simulink library "AeroLib"  (Simulink 6.0)
settings: Solver=ode45  SolverMode=SingleTasking  StartTime=0.0  StopTime=10.0  RelTol=1e-3
undefined symbols (not defined in the file): Aero, Ap, Atm, Control, Controls, Eng, Flight_cg, Flight_DamperON, Flight_delta_isa, Flight_DeltaSpiral, Flight_InertiaSelect, Flight_ixx, Flight_ixz, Flight_iyy, Flight_izz, Flight_latitude, Flight_LoiterLenght, Flight_LoiterMode, Flight_LoiterRadius, Flight_longitude, Flight_MaxTargetPoints, Flight_SensorsON, Flight_TimeStep, Flight_TowerWind_X, Flight_TowerWind_Y, Flight_TowerWind_Z, Flight_TowerWindON, Flight_Trimming, Flight_TurbON, Flight_weight, Flight_WindGustON, Flight_WindShearON, Flight_ycg, Flight_zcg, Geom, Lgear, Mass, PEG_CDwbnp, PEG_CLht, PEG_CLht_elev, PEG_CLwbnp, PEG_CMht, PEG_CMwbnp, PEG_CNbeta, PEG_CNr, PEG_CNrud, PEG_CRail, PEG_CRbeta, PEG_CRp, PEG_CRrud, PEG_CYbeta, PEG_CYrud, pow, Sensors
libraries: AeroLib x133, simulink3 x49, simulink x37, aerospace x11
(part 2 of 7)

== system AeroLib/AtmosphericData/Simple_Wind_Gust ==
  note: Horizontal wind direction 0 deg ==> North
      | Horizontal wind direction 90 deg ==> East
      | Horizontal wind direction 180 deg ==> South
      | Horizontal wind direction 270 deg ==> West
      |
      |
      |
      |
      |
      |
      |
      |
      |
      |
      |
      |
      |
      |
      |
      | Vertical wind speed negative ==> Up (ft/s)
      | Vertical wind speed positive ==> Down (ft/s)
  From_Reset : Inport  Port=1  LatchInput=off
  From_Inputs : Inport  Port=2  LatchInput=off
  Band-Limited White Noise : simulink3/Sources/Band-Limited White Noise  Cov=[0.1]  Ts=Flight_TimeStep  seed=[23341]
  Bus Selector : BusSelector  DialogController=Simulink.DDGSource_Bus  OutputSignals=Horiz_Wind_Speed,Horiz_Wind_Dir,Vert_Wind_Speed
  Constant2 : Constant  Value=Flight_WindGustON
  Deg-->Rad : Gain  Gain=pi/180  SaturateOnIntegerOverflow=on
  Demux : Demux  Outputs=2
  Gain : Gain  Gain=Wgain  SaturateOnIntegerOverflow=on
  Mux : Mux  Inputs=2
  Mux1 : Mux  Inputs=3
  Product : Product  SaturateOnIntegerOverflow=on  InputSameDT=on
  Product1 : Product  SaturateOnIntegerOverflow=on  InputSameDT=on
  Stateless_Integrator : AeroLib/AMS_StatelessFilters/Stateless_Integrator
  Sum : Sum  Inputs=|++  SaturateOnIntegerOverflow=on  InputSameDT=on
  Trigonometric Function : Trigonometry  Operator=cos
  Trigonometric Function1 : Trigonometry
  WindGust : TransferFcn  Numerator=WGfac/sqrt(F^3)*[sqrt(3)*F,1]  Denominator=[1 (2/F) 1/F^2]
  Xo : Constant  Value=0
  fps-->mps : Gain  Gain=0.3048  SaturateOnIntegerOverflow=on
  kt-->mps : Gain  Gain=0.5144444  SaturateOnIntegerOverflow=on
  Wind_mps : Outport
  wires:
  Bus Selector/2 -> Deg-->Rad/1  "<Horiz_Wind_Dir>"
  Deg-->Rad/1 -> Trigonometric Function/1, Trigonometric Function1/1
  Trigonometric Function/1 -> Mux/1
  Trigonometric Function1/1 -> Mux/2
  Mux/1 -> Product/2
  Bus Selector/1 -> kt-->mps/1  "<Horiz_Wind_Speed>"
  Band-Limited White Noise/1 -> WindGust/1
  WindGust/1 -> Gain/1
  Gain/1 -> Stateless_Integrator/3  "WingZ"
  Product/1 -> Demux/1
  Demux/1 -> Mux1/1
  Demux/2 -> Mux1/2
  Mux1/1 -> Wind_mps/1
  kt-->mps/1 -> Product/1
  Stateless_Integrator/1 -> Product1/1
  Constant2/1 -> Product1/2
  From_Reset/1 -> Stateless_Integrator/1
  Xo/1 -> Stateless_Integrator/2
  From_Inputs/1 -> Bus Selector/1
  Bus Selector/3 -> fps-->mps/1  "<Vert_Wind_Speed>"
  fps-->mps/1 -> Sum/1
  Product1/1 -> Sum/2
  Sum/1 -> Mux1/3

== system AeroLib/Autopilot/AutoPilot_Out ==
  Bus Creator1 : BusCreator  DialogController=Simulink.DDGSource_Bus  Inputs=10
  Constant : Constant  Value=[0 0 0 0 0 0 0 0]
  Constant5 : Constant  Value=0
  Constant6 : Constant  Value=0
  Demux1 : Demux  Outputs=8
  AP_Out : Outport
  wires:
  Demux1/6 -> Bus Creator1/6  "Bearing"
  Demux1/5 -> Bus Creator1/5  "Throttle_RH_cmd"
  Demux1/4 -> Bus Creator1/4  "Throttle_LH_cmd"
  Demux1/3 -> Bus Creator1/3  "Rudder_cmd"
  Demux1/2 -> Bus Creator1/2  "Aileron_cmd"
  Demux1/1 -> Bus Creator1/1  "Elevator_cmd"
  Demux1/7 -> Bus Creator1/7  "Time_to_Go"
  Demux1/8 -> Bus Creator1/8  "Point_N"
  Constant5/1 -> Bus Creator1/9  "AP_Brake"
  Constant6/1 -> Bus Creator1/10  "AP_Caster"
  Constant/1 -> Demux1/1
  Bus Creator1/1 -> AP_Out/1

== system AeroLib/Autopilot/Autopilot ==
  From_FSC : Inport  Port=1  LatchInput=off
  From_Inputs : Inport  Port=2  LatchInput=off
  From_Reset : Inport  Port=3  LatchInput=off
  From_Prop : Inport  Port=4  LatchInput=off
  AutopilotEngage : Subsystem
  Bus Creator : BusCreator  DialogController=Simulink.DDGSource_Bus  Inputs=10
  Constant1 : Constant  Value=0
  Constant2 : Constant  Value=0
  Constant3 : Constant  Value=[0 0 0 0 0]
  Dampers : Subsystem
  Demux1 : Demux  Outputs=8
  Guidance : Subsystem
  Mux1 : Mux  Inputs=8
  Mux2 : Mux
  PID_AutoPilot : Subsystem
  Product : Product  SaturateOnIntegerOverflow=on  InputSameDT=on
  Sum4 : Sum  SaturateOnIntegerOverflow=on  InputSameDT=on
  TargetPointsTransform : Subsystem
  AP_Out : Outport
  wires:
  AutopilotEngage/1(AutopilotON) -> Product/2
  From_Prop/1 -> AutopilotEngage/2(From_Prop), Guidance/4(From_Prop), Dampers/3(From_Prop)
  Guidance/3(Alt_Err) -> PID_AutoPilot/3(Alt_Err)
  Constant2/1 -> Bus Creator/10  "AP_Caster"
  Constant1/1 -> Bus Creator/9  "AP_Brake"
  From_Reset/1 -> Guidance/5(From_Reset), PID_AutoPilot/4(From_Reset), Dampers/1(From_Reset)
  Demux1/8 -> Bus Creator/8  "Point_N"
  Guidance/6(Point_N) -> Mux1/8
  TargetPointsTransform/1(TP_XY) -> Guidance/1(PointsXY)
  Product/1 -> Sum4/2
  Mux1/1 -> Product/1
  PID_AutoPilot/1(Elev_cmd) -> Mux1/1
  PID_AutoPilot/2(Ail_cmd) -> Mux1/2
  PID_AutoPilot/3(Rud_cmd) -> Mux1/3
  PID_AutoPilot/4(Thr_LH_cmd) -> Mux1/4
  PID_AutoPilot/5(Thr_RH_cmd) -> Mux1/5
  From_FSC/1 -> AutopilotEngage/3(From_FSC), PID_AutoPilot/5(From_Sen), Guidance/3(From_FSC), Dampers/2(From_Sen)
  Guidance/1(Speed_Err) -> PID_AutoPilot/1(Speed_Err)
  From_Inputs/1 -> AutopilotEngage/1(From_Inputs), Guidance/6(From_Inputs), Dampers/4(From_Inputs), TargetPointsTransform/1(From_Inputs)
  Guidance/4(Bearing) -> Mux1/6
  Guidance/5(Time_to_Go) -> Mux1/7
  Bus Creator/1 -> AP_Out/1
  Demux1/7 -> Bus Creator/7  "Time_to_Go"
  Demux1/1 -> Bus Creator/1  "Elevator_cmd"
  Demux1/2 -> Bus Creator/2  "Aileron_cmd"
  Demux1/3 -> Bus Creator/3  "Rudder_cmd"
  Demux1/4 -> Bus Creator/4  "Throttle_LH_cmd"
  Demux1/5 -> Bus Creator/5  "Throttle_RH_cmd"
  Demux1/6 -> Bus Creator/6  "Bearing"
  Guidance/2(Track_Err) -> PID_AutoPilot/2(Track_err)
  TargetPointsTransform/2(TP_Lat_Lon) -> Guidance/2(PointsLatLon)
  Sum4/1 -> Demux1/1
  Dampers/1(Elev_cmd) -> Mux2/1
  Dampers/2(Ail_cmd) -> Mux2/2
  Dampers/3(Rud_cmd) -> Mux2/3
  Constant3/1 -> Mux2/4
  Mux2/1 -> Sum4/1

== system AeroLib/Autopilot/Counter_Point ==
  Input_Param : Inport  Port=1  LatchInput=off
  From_Reset : Inport  Port=2  LatchInput=off
  Bus Selector : BusSelector  DialogController=Simulink.DDGSource_Bus  OutputSignals=TimeStep
  Clock4 : Clock
      settings: Decimation=10
  Fcn : Fcn  Expr=u < MinDist
  Fcn2 : Fcn  Expr=u == 0
  Logical Operator : Logic
  Mem : Memory
  Memory : Memory  Orientation=left
  Mux : Mux  Inputs=2
  Next_Step : Fcn  Expr=u(2) < u(1)*1.5
  Sum : Sum  Inputs=|++  SaturateOnIntegerOverflow=on  InputSameDT=on
  Sum1 : Sum  Inputs=|+-  SaturateOnIntegerOverflow=on  InputSameDT=on
  Sw4 : Switch  Threshold=0.5  SaturateOnIntegerOverflow=on  InputSameDT=on
  Point_N : Outport
  wires:
  Fcn/1 -> Fcn2/1, Logical Operator/2
  Fcn2/1 -> Sw4/2
  Sw4/1 -> Mem/1, Sum1/2
  Mem/1 -> Sw4/3
  Clock4/1 -> Sum1/1, Sw4/1
  Sum/1 -> Memory/1, Point_N/1
  Memory/1 -> Sum/2
  Next_Step/1 -> Logical Operator/1
  Logical Operator/1 -> Sum/1
  Input_Param/1 -> Fcn/1
  From_Reset/1 -> Bus Selector/1
  Sum1/1 -> Mux/2
  Mux/1 -> Next_Step/1
  Bus Selector/1 -> Mux/1  "<TimeStep>"

== system AeroLib/Autopilot/GeodCoor to XY ==
  Lat_cmd : Inport  Port=1  LatchInput=off
  Long_cmd : Inport  Port=2  LatchInput=off
  Alt_cmd : Inport  Port=3  LatchInput=off
  Deg-->Rad : Gain  Gain=pi/180  SaturateOnIntegerOverflow=on
  Deg-->Rad1 : Gain  Gain=pi/180  SaturateOnIntegerOverflow=on
  Geo2orto : Subsystem
  ft-->m : Gain  Gain=0.3048  SaturateOnIntegerOverflow=on
  X_dist : Outport
  Y_dist : Outport  Port=2
  PresAlt : Outport  Port=3
  wires:
  Long_cmd/1 -> Deg-->Rad1/1
  Alt_cmd/1 -> ft-->m/1
  Lat_cmd/1 -> Deg-->Rad/1
  ft-->m/1 -> PresAlt/1, Geo2orto/3(Alt_In)
  Geo2orto/1(X_m) -> X_dist/1
  Geo2orto/2(Y_m) -> Y_dist/1
  Deg-->Rad1/1 -> Geo2orto/2(Lon_In)
  Deg-->Rad/1 -> Geo2orto/1(Lat_In)

== system AeroLib/Autopilot/Geod_Target_Errors ==
  Lat_req : Inport  Port=1  LatchInput=off
  Lon_req : Inport  Port=2  LatchInput=off
  Speed_Req : Inport  Port=3  LatchInput=off
  From_FSC : Inport  Port=4  LatchInput=off
  Alt_req : Inport  Port=5  LatchInput=off
  Bus Selector1 : BusSelector  DialogController=Simulink.DDGSource_Bus  OutputSignals=FSC_Latitude_deg,FSC_Longitude_deg,FSC_Altitude_ft,FSC_TrackMag_deg,FSC_GrSpeed_kt
  Bus Selector3 : BusSelector  DialogController=Simulink.DDGSource_Bus  OutputSignals=FSC_Altitude_ft,IRU_RadarAlt_ft
  Product : Product  Inputs=*/  SaturateOnIntegerOverflow=on  InputSameDT=on
  Subsystem : Subsystem
  Sum1 : Sum  Inputs=-+|  SaturateOnIntegerOverflow=on  InputSameDT=on
  Sum4 : Sum  Inputs=+-  SaturateOnIntegerOverflow=on  InputSameDT=on
  Sum5 : Sum  Inputs=+-  SaturateOnIntegerOverflow=on  InputSameDT=on
  Switch1 : Switch  Threshold=3000  SaturateOnIntegerOverflow=on  InputSameDT=on
  ft--->m : Gain  Gain=0.3048  SaturateOnIntegerOverflow=on
  kt--->mps : Gain  Gain=0.5144444  SaturateOnIntegerOverflow=on
  Distance_m : Outport
  Time_to_Go : Outport  Port=2
  Track_Err : Outport  Port=3
  Speed_Err : Outport  Port=4
  Bearing : Outport  Port=5
  Alt_Err : Outport  Port=6
  wires:
  Sum5/1 -> Alt_Err/1
  Alt_req/1 -> Sum5/1
  ft--->m/1 -> Sum5/2
  Switch1/1 -> ft--->m/1
  Bus Selector3/2 -> Switch1/3, Switch1/2  "<IRU_RadarAlt_ft>"
  Bus Selector3/1 -> Switch1/1  "<FSC_Altitude_ft>"
  Sum4/1 -> Track_Err/1
  From_FSC/1 -> Bus Selector3/1, Bus Selector1/1
  Bus Selector1/4 -> Sum4/2  "<FSC_TrackMag_deg>"
  Bus Selector1/2 -> Subsystem/4(Lon)  "<FSC_Longitude_deg>"
  Bus Selector1/1 -> Subsystem/3(Lat)  "<FSC_Latitude_deg>"
  Bus Selector1/5 -> kt--->mps/1, Sum1/1  "<FSC_GrSpeed_kt>"
  Subsystem/2(Bearing_Deg) -> Bearing/1, Sum4/1
  kt--->mps/1 -> Product/2
  Sum1/1 -> Speed_Err/1
  Speed_Req/1 -> Sum1/2
  Product/1 -> Time_to_Go/1
  Lon_req/1 -> Subsystem/2(Lon_Req)
  Lat_req/1 -> Subsystem/1(Lat_Req)
  Subsystem/1(Distance_m) -> Product/1, Distance_m/1
  Bus Selector1/3 -> Subsystem/5(Alt_ft)  "<FSC_Altitude_ft>"

== system AeroLib/Autopilot/PID ==
  From_Reset : Inport  Port=1  LatchInput=off
  Err : Inport  Port=2  LatchInput=off
  CommandSaturation : Saturate  UpperLimit=Lim_Com  LowerLimit=-Lim_Com
  DerGain : Gain  Gain=D  SaturateOnIntegerOverflow=on
  ErrorSaturation : Saturate  UpperLimit=Lim_Err  LowerLimit=-Lim_Err
  Fcn : Fcn  Expr=abs(u) < Lim_I
  IntGain : Gain  Gain=I  SaturateOnIntegerOverflow=on
  Product : Product  SaturateOnIntegerOverflow=on
  PropGain : Gain  Gain=P  SaturateOnIntegerOverflow=on
  Stateless_HighPass1 : AeroLib/AMS_StatelessFilters/Stateless_HighPass
  Stateless_Integrator : AeroLib/AMS_StatelessFilters/Stateless_Integrator
  Sum : Sum  Inputs=+++  SaturateOnIntegerOverflow=on  InputSameDT=on
  Tau : Constant  Value=10
  Xo : Constant  Value=0
  Cmd : Outport  InitialOutput=0
  wires:
  Fcn/1 -> Product/1
  ErrorSaturation/1 -> Stateless_HighPass1/2, Product/2, PropGain/1
  CommandSaturation/1 -> Cmd/1
  Sum/1 -> CommandSaturation/1
  IntGain/1 -> Sum/2
  PropGain/1 -> Sum/1
  Stateless_Integrator/1 -> IntGain/1
  Err/1 -> ErrorSaturation/1, Fcn/1
  Xo/1 -> Stateless_Integrator/2
  From_Reset/1 -> Stateless_Integrator/1, Stateless_HighPass1/1
  Tau/1 -> Stateless_HighPass1/3
  Stateless_HighPass1/1 -> DerGain/1
  Product/1 -> Stateless_Integrator/3
  DerGain/1 -> Sum/3

== system AeroLib/Autopilot/Target_Errors ==
  Y_req : Inport  Port=1  LatchInput=off
  X_req : Inport  Port=2  LatchInput=off
  Speed_Req : Inport  Port=3  LatchInput=off
  From_FSC : Inport  Port=4  LatchInput=off
  Alt_req : Inport  Port=5  LatchInput=off
  Bus Selector1 : BusSelector  DialogController=Simulink.DDGSource_Bus  OutputSignals=FSC_Xdist_m,FSC_Ydist_m,FSC_TrackMag_deg,FSC_GrSpeed_kt
  Bus Selector3 : BusSelector  DialogController=Simulink.DDGSource_Bus  OutputSignals=FSC_Altitude_ft,IRU_RadarAlt_ft
  Mux : Mux  Inputs=2
  Product : Product  Inputs=*/  SaturateOnIntegerOverflow=on  InputSameDT=on
  Sum1 : Sum  Inputs=-+|  SaturateOnIntegerOverflow=on  InputSameDT=on
  Sum2 : Sum  Inputs=|+-  SaturateOnIntegerOverflow=on  InputSameDT=on
  Sum3 : Sum  Inputs=|+-  SaturateOnIntegerOverflow=on  InputSameDT=on
  Sum4 : Sum  Inputs=+-  SaturateOnIntegerOverflow=on  InputSameDT=on
  Sum5 : Sum  Inputs=+-  SaturateOnIntegerOverflow=on  InputSameDT=on
  Switch1 : Switch  Threshold=3000  SaturateOnIntegerOverflow=on  InputSameDT=on
  Trigonometric Function : Trigonometry  Operator=atan2
  dist : Fcn  Expr=sqrt( u(1)*u(1) + u(2)*u(2) )
  ft--->m : Gain  Gain=0.3048  SaturateOnIntegerOverflow=on
  kt--->mps : Gain  Gain=0.5144444  SaturateOnIntegerOverflow=on
  rad--->deg : Gain  Gain=180/pi  SaturateOnIntegerOverflow=on
  Distance : Outport
  Time_to_Go : Outport  Port=2
  Track_Err : Outport  Port=3
  Speed_Err : Outport  Port=4
  Bearing : Outport  Port=5
  Alt_Err : Outport  Port=6
  wires:
  Product/1 -> Time_to_Go/1
  Speed_Req/1 -> Sum1/2
  X_req/1 -> Sum2/1
  Y_req/1 -> Sum3/1
  Sum1/1 -> Speed_Err/1
  kt--->mps/1 -> Product/2
  rad--->deg/1 -> Sum4/1, Bearing/1
  Bus Selector1/4 -> Sum1/1, kt--->mps/1  "<FSC_GrSpeed_kt>"
  Bus Selector1/1 -> Sum2/2  "<FSC_Xdist_m>"
  Bus Selector1/2 -> Sum3/2  "<FSC_Ydist_m>"
  Sum3/1 -> Trigonometric Function/1, Mux/1
  Sum2/1 -> Trigonometric Function/2, Mux/2
  Mux/1 -> dist/1
  dist/1 -> Distance/1, Product/1
  Bus Selector1/3 -> Sum4/2  "<FSC_TrackMag_deg>"
  Trigonometric Function/1 -> rad--->deg/1
  From_FSC/1 -> Bus Selector1/1, Bus Selector3/1
  Sum4/1 -> Track_Err/1
  Bus Selector3/1 -> Switch1/1, Switch1/2  "<FSC_Altitude_ft>"
  Bus Selector3/2 -> Switch1/3  "<IRU_RadarAlt_ft>"
  Switch1/1 -> ft--->m/1
  ft--->m/1 -> Sum5/2
  Alt_req/1 -> Sum5/1
  Sum5/1 -> Alt_Err/1

== system AeroLib/Controls/Simple_Aileron_Actuator ==
  AilCmd : Inport  Port=1  LatchInput=off
  Aileron_LH : Integrator  LimitOutput=on  UpperSaturationLimit=up/2  LowerSaturationLimit=low/2
  Aileron_RH : Integrator  LimitOutput=on  UpperSaturationLimit=up/2  LowerSaturationLimit=low/2
  Demux : Demux  Outputs=2
  Fcn2 : Fcn  Expr=u(2)-u(1)
  FlightTrim_Switch : AeroLib/AMS_StatelessFilters/FlightTrim_Switch
  FlightTrim_Switch1 : AeroLib/AMS_StatelessFilters/FlightTrim_Switch
  Gain1 : Gain  Gain=Control.Wheel.Ratio(2)  SaturateOnIntegerOverflow=on
  Gain2 : Gain  Gain=Control.Wheel.Ratio(1)  SaturateOnIntegerOverflow=on
  Gain3 : Gain  Gain=-Control.Wheel.Ratio(2)  SaturateOnIntegerOverflow=on
  Gain4 : Gain  Gain=tau  SaturateOnIntegerOverflow=on
  Gain5 : Gain  Gain=tau  SaturateOnIntegerOverflow=on
  Left : Gain  Gain=-Control.Wheel.Ratio(1)  SaturateOnIntegerOverflow=on
  Mux : Mux  Inputs=2
  Mux1 : Mux  Inputs=2
  Mux2 : Mux  Inputs=2
  Saturation : Saturate  UpperLimit=up  LowerLimit=low
  Sum : Sum  Inputs=|+-  SaturateOnIntegerOverflow=on  InputSameDT=on
  Sum1 : Sum  Inputs=|+-  SaturateOnIntegerOverflow=on  InputSameDT=on
  Switch : Switch  SaturateOnIntegerOverflow=on  InputSameDT=on
  Ail_deg : Outport
  wires:
  FlightTrim_Switch/1 -> Gain5/1
  FlightTrim_Switch1/1 -> Gain4/1
  Sum/1 -> FlightTrim_Switch1/1  "err"
  Gain4/1 -> Aileron_LH/1
  Aileron_LH/1 -> Sum/2, Mux/1  "Stab"
  Sum1/1 -> FlightTrim_Switch/1  "err"
  Gain5/1 -> Aileron_RH/1
  Aileron_RH/1 -> Mux/2, Sum1/2  "Stab"
  Mux/1 -> Fcn2/1
  Fcn2/1 -> Saturation/1
  Mux2/1 -> Switch/3
  Mux1/1 -> Switch/1
  Gain2/1 -> Mux2/2  "Ail_RH"
  Gain3/1 -> Mux2/1  "Ail_LH"
  Left/1 -> Mux1/1  "Ail_LH"
  Gain1/1 -> Mux1/2  "Ail_RH"
  Switch/1 -> Demux/1
  Demux/1 -> Sum/1
  Demux/2 -> Sum1/1
  AilCmd/1 -> Switch/2, Gain3/1, Gain2/1, Gain1/1, Left/1
  Saturation/1 -> Ail_deg/1

== system AeroLib/Controls/Simple_Controls ==
  From_AP : Inport  Port=1  LatchInput=off
  From_Inputs : Inport  Port=2  LatchInput=off
  From_Reset : Inport  Port=3  LatchInput=off
  Bus Creator : BusCreator  DialogController=Simulink.DDGSource_Bus  Inputs=7
  Bus Selector : BusSelector  DialogController=Simulink.DDGSource_Bus  OutputSignals=Elevator_cmd,Aileron_cmd,Rudder_cmd,Throttle_LH_cmd,Throttle_RH_cmd
  Bus Selector1 : BusSelector  DialogController=Simulink.DDGSource_Bus  OutputSignals=Column,Wheel,Pedal,Throttle_LH,Throttle_RH,FlapSlatLever,TrimCmd
  Gain : Gain  Gain=-1  SaturateOnIntegerOverflow=on
  Gain1 : Gain  Gain=-1  SaturateOnIntegerOverflow=on
  Simple_Aileron_Actuator : AeroLib/Controls/Simple_Aileron_Actuator  tau=Controls.Ail.Gain  ratio=Control.Wheel.Ratio  up=Controls.Ail.MaxAngle  low=-Controls.Ail.MaxAngle
  Simple_Elevator_Actuator : AeroLib/Controls/Simple_Elevator_Actuator  tau=Controls.Elev.Gain  up=Controls.Elev.MaxPos  low=Controls.Elev.MaxNeg
  Simple_Flap_Actuator : AeroLib/Controls/Simple_Flap_Actuator  flap_pos=Controls.flapslat  flap_defl=Controls.flap.Defl  flap_rate=Controls.flap.Rate
  Simple_Rudder_Actuator : AeroLib/Controls/Simple_Rudder_Actuator  tau=Controls.Rudder.Gain  up=Controls.Rudder.MaxAngle  low=-Controls.Rudder.MaxAngle
  Simple_Stab_Actuator : AeroLib/Controls/Simple_Stab_Actuator  gain=Controls.Stab.Gain
  Sum{,1..4} (5 alike) : Sum  Inputs=|++  SaturateOnIntegerOverflow=on  InputSameDT=on
  Ctrl_Out : Outport
  wires:
  From_Reset/1 -> Simple_Flap_Actuator/2
  Bus Selector/5 -> Sum4/1  "<Throttle_RH_cmd>"
  Sum4/1 -> Bus Creator/5  "Thr_RH"
  Sum3/1 -> Bus Creator/4  "Thr_LH"
  Bus Selector/4 -> Sum3/1  "<Throttle_LH_cmd>"
  Simple_Stab_Actuator/1 -> Bus Creator/7  "Stab_deg"
  Simple_Flap_Actuator/1 -> Bus Creator/6  "Flap_deg"
  Bus Selector/3 -> Sum2/1  "<Rudder_cmd>"
  Sum2/1 -> Gain1/1
  Sum1/1 -> Simple_Aileron_Actuator/1
  Bus Selector/2 -> Sum1/1  "<Aileron_cmd>"
  Sum/1 -> Gain/1
  Bus Selector/1 -> Sum/1  "<Elevator_cmd>"
  Bus Selector1/5 -> Sum4/2  "<Throttle_RH>"
  Bus Selector1/4 -> Sum3/2  "<Throttle_LH>"
  Bus Selector1/7 -> Simple_Stab_Actuator/1  "<TrimCmd>"
  Bus Selector1/6 -> Simple_Flap_Actuator/1  "<FlapSlatLever>"
  Bus Selector1/3 -> Sum2/2  "<Pedal>"
  Bus Selector1/2 -> Sum1/2  "<Wheel>"
  Bus Selector1/1 -> Sum/2  "<Column>"
  From_Inputs/1 -> Bus Selector1/1
  Simple_Aileron_Actuator/1 -> Bus Creator/2  "Ail_deg"
  Simple_Elevator_Actuator/1 -> Bus Creator/1  "Elev_deg"
  Simple_Rudder_Actuator/1 -> Bus Creator/3  "Rud_deg"
  Bus Creator/1 -> Ctrl_Out/1
  From_AP/1 -> Bus Selector/1
  Gain/1 -> Simple_Elevator_Actuator/1
  Gain1/1 -> Simple_Rudder_Actuator/1

== system AeroLib/Controls/Simple_Elevator_Actuator ==
  ElevCmd : Inport  Port=1  LatchInput=off
  Elevator : Integrator  LimitOutput=on  UpperSaturationLimit=up  LowerSaturationLimit=low
  FlightTrim_Switch : AeroLib/AMS_StatelessFilters/FlightTrim_Switch
  Gain_Amp : Gain  Gain=tau  SaturateOnIntegerOverflow=on
  Sum : Sum  Inputs=|+-  SaturateOnIntegerOverflow=on  InputSameDT=on
  Elev_deg : Outport
  wires:
  FlightTrim_Switch/1 -> Gain_Amp/1
  Gain_Amp/1 -> Elevator/1
  ElevCmd/1 -> Sum/1
  Elevator/1 -> Sum/2, Elev_deg/1  "Stab"
  Sum/1 -> FlightTrim_Switch/1  "err"

== system AeroLib/Controls/Simple_Flap_Actuator ==
  FSLever : Inport  Port=1  LatchInput=off
  From_Reset : Inport  Port=2  LatchInput=off
  Fcn : Fcn  Expr=(u(1)+u(2))/2
  FlapPos : Lookup  DialogController=Simulink.DDGSource  InputValues=flap_pos  OutputValues=flap_defl  SaturateOnIntegerOverflow=on
  Max : Constant  Value=Controls.flap.Defl(max(size(Controls.flap.Defl)))
  Max1 : Constant  Value=Controls.flap.Defl(max(size(Controls.flap.Defl)))
  Min : Constant  Value=0
  Min1 : Constant  Value=0
  Mux : Mux  Inputs=2
  RateLimits : Subsystem
  Stateless_LimIntegrator : AeroLib/AMS_StatelessFilters/Stateless_LimIntegrator
  Stateless_LimIntegrator1 : AeroLib/AMS_StatelessFilters/Stateless_LimIntegrator
  Sum : Sum  Inputs=|+-  SaturateOnIntegerOverflow=on  InputSameDT=on
  Sum1 : Sum  Inputs=|+-  SaturateOnIntegerOverflow=on  InputSameDT=on
  Variable Limiter : Subsystem
  Variable Limiter1 : Subsystem
  freq_LH : Gain  Gain=10  SaturateOnIntegerOverflow=on
  freq_RH : Gain  Gain=10  SaturateOnIntegerOverflow=on
  Flap_deg : Outport
  wires:
  Stateless_LimIntegrator1/1 -> Sum/2, Mux/2  "rhflap"
  Stateless_LimIntegrator/1 -> Mux/1, Sum1/2  "lhflap"
  Sum1/1 -> freq_LH/1
  Variable Limiter/1(SigSat) -> Stateless_LimIntegrator/3
  Sum/1 -> freq_RH/1
  Variable Limiter1/1(SigSat) -> Stateless_LimIntegrator1/3
  freq_LH/1 -> Variable Limiter/1(Sig)
  freq_RH/1 -> Variable Limiter1/1(Sig)
  FlapPos/1 -> Sum1/1, Stateless_LimIntegrator/2, Sum/1, Stateless_LimIntegrator1/2  "Cmd"
  Max/1 -> Stateless_LimIntegrator/5
  Min/1 -> Stateless_LimIntegrator/4
  Max1/1 -> Stateless_LimIntegrator1/5
  Min1/1 -> Stateless_LimIntegrator1/4
  FSLever/1 -> RateLimits/1(FSLever), FlapPos/1
  RateLimits/1(FlapRate) -> Variable Limiter/2(Sat), Variable Limiter1/2(Sat)
  Mux/1 -> Fcn/1
  Fcn/1 -> Flap_deg/1
  From_Reset/1 -> Stateless_LimIntegrator/1, Stateless_LimIntegrator1/1

== system AeroLib/Controls/Simple_Rudder_Actuator ==
  RudCmd : Inport  Port=1  LatchInput=off
  FlightTrim_Switch : AeroLib/AMS_StatelessFilters/FlightTrim_Switch
  Gain_Amp : Gain  Gain=tau  SaturateOnIntegerOverflow=on
  Rudder : Integrator  LimitOutput=on  UpperSaturationLimit=up  LowerSaturationLimit=low
  Sum : Sum  Inputs=|+-  SaturateOnIntegerOverflow=on  InputSameDT=on
  Rud_deg : Outport
  wires:
  FlightTrim_Switch/1 -> Gain_Amp/1
  RudCmd/1 -> Sum/1
  Rudder/1 -> Sum/2, Rud_deg/1  "Stab"
  Gain_Amp/1 -> Rudder/1
  Sum/1 -> FlightTrim_Switch/1  "err"

== system AeroLib/Controls/Simple_Stab_Actuator ==
  TrimCmd : Inport  Port=1  LatchInput=off
  Gain4 : Gain  Gain=gain  SaturateOnIntegerOverflow=on
  Stab : Integrator  LimitOutput=on  UpperSaturationLimit=up  LowerSaturationLimit=low
  Stab_deg : Outport
  wires:
  Stab/1 -> Stab_deg/1
  Gain4/1 -> Stab/1
  TrimCmd/1 -> Gain4/1

== system AeroLib/CoordinateSystems/BOA2LEF ==
  note: Transformation from
      | Body Axes to
      | Local Earth Frame
  Body_In : Inport  Port=1  LatchInput=off
  DCM : Inport  Port=2  LatchInput=off
  Product : Product  Multiplication=Matrix(*)  SaturateOnIntegerOverflow=on  InputSameDT=on
  Earth_Out : Outport  InitialOutput=0
  wires:
  DCM/1 -> Product/1
  Body_In/1 -> Product/2
  Product/1 -> Earth_Out/1

== system AeroLib/CoordinateSystems/EUL2DCM ==
  note: Directional Cosine Matrix
      |
      | "1-2-3" rotation matrix
      | From Euler Angles (phi, theta, psi)
  Euler : Inport  Port=1  LatchInput=off
  Mux2 : Mux  Inputs=9
  Reshape : simulink3/Signals & Systems/Reshape  OutputDimensionality=Customize  OutputDimensions=[3,3]
  _1_1 : Fcn  Expr=cos(u[3])*cos(u[2])
  _1_2 : Fcn  Expr=sin(u[3])*cos(u[2])
  _1_3 : Fcn  Expr=-sin(u[2])
  _2_1 : Fcn  Expr=cos(u[3])*sin(u[2])*sin(u[1])-sin(u[3])*cos(u[1])
  _2_2 : Fcn  Expr=sin(u[3])*sin(u[2])*sin(u[1])+cos(u[3])*cos(u[1])
  _2_3 : Fcn  Expr=cos(u[2])*sin(u[1])
  _3_1 : Fcn  Expr=cos(u[3])*sin(u[2])*cos(u[1])+sin(u[3])*sin(u[1])
  _3_2 : Fcn  Expr=sin(u[3])*sin(u[2])*cos(u[1])-cos(u[3])*sin(u[1])
  _3_3 : Fcn  Expr=cos(u[2])*cos(u[1])
  DCM : Outport
  wires:
  Reshape/1 -> DCM/1
  Euler/1 -> _1_1/1, _3_3/1, _3_2/1, _3_1/1, _2_3/1, _2_2/1, _2_1/1, _1_3/1, _1_2/1
  Mux2/1 -> Reshape/1
  _1_1/1 -> Mux2/1
  _1_2/1 -> Mux2/2
  _1_3/1 -> Mux2/3
  _2_1/1 -> Mux2/4
  _2_2/1 -> Mux2/5
  _2_3/1 -> Mux2/6
  _3_1/1 -> Mux2/7
  _3_2/1 -> Mux2/8
  _3_3/1 -> Mux2/9

== system AeroLib/CoordinateSystems/EUL2QUA ==
  note: Rotation representation
      |
      | Euler angles (rad) to
      | Quaternion parameters
  Euler : Inport  Port=1  LatchInput=off
  Gain : Gain  Gain=0.5  SaturateOnIntegerOverflow=on
  Mux : Mux
  q1 : Fcn  Expr=cos(u(3))*cos(u(2))*cos(u(1)) + sin(u(3))*sin(u(2))*sin(u(1))
  q2 : Fcn  Expr=cos(u(3))*cos(u(2))*sin(u(1)) - sin(u(3))*sin(u(2))*cos(u(1))
  q3 : Fcn  Expr=cos(u(3))*sin(u(2))*cos(u(1)) + sin(u(3))*cos(u(2))*sin(u(1))
  q4 : Fcn  Expr=sin(u(3))*cos(u(2))*cos(u(1)) - cos(u(3))*sin(u(2))*sin(u(1))
  Quaternion : Outport
  wires:
  Euler/1 -> Gain/1
  q1/1 -> Mux/1
  q2/1 -> Mux/2
  q3/1 -> Mux/3
  q4/1 -> Mux/4
  Gain/1 -> q2/1, q1/1, q3/1, q4/1
  Mux/1 -> Quaternion/1

== system AeroLib/CoordinateSystems/QUA2DCM ==
  note: Directional Cosine Matrix
      |
      | "1-2-3" rotation matrix
      | from Quaternion parameters
  Quaternion : Inport  Port=1  LatchInput=off
  Mux2 : Mux  Inputs=9
  Reshape : simulink3/Signals & Systems/Reshape  OutputDimensionality=Customize  OutputDimensions=[3,3]
  _1_1 : Fcn  Expr=pow(u[1],2)+pow(u[2],2)-pow(u[3],2)-pow(u[4],2)
  _1_2 : Fcn  Expr=2*(u[2]*u[3] + u[1]*u[4])
  _1_3 : Fcn  Expr=2*(u[2]*u[4]-u[1]*u[3])
  _2_1 : Fcn  Expr=2*(u[2]*u[3]-u[1]*u[4])
  _2_2 : Fcn  Expr=pow(u[1],2)-pow(u[2],2)+pow(u[3],2)-pow(u[4],2)
  _2_3 : Fcn  Expr=2*(u[3]*u[4]+u[1]*u[2])
  _3_1 : Fcn  Expr=2*(u[1]*u[3]+u[2]*u[4])
  _3_2 : Fcn  Expr=2*(u[3]*u[4]-u[1]*u[2])
  _3_3 : Fcn  Expr=pow(u[1],2)-pow(u[2],2)-pow(u[3],2)+pow(u[4],2)
  DCM : Outport  InitialOutput=0
  wires:
  _3_3/1 -> Mux2/9
  _3_2/1 -> Mux2/8
  _3_1/1 -> Mux2/7
  _2_3/1 -> Mux2/6
  _2_2/1 -> Mux2/5
  _2_1/1 -> Mux2/4
  _1_3/1 -> Mux2/3
  _1_2/1 -> Mux2/2
  _1_1/1 -> Mux2/1
  Mux2/1 -> Reshape/1
  Reshape/1 -> DCM/1
  Quaternion/1 -> _3_2/1, _3_3/1, _3_1/1, _2_3/1, _2_1/1, _1_3/1, _1_2/1, _1_1/1, _2_2/1

== system AeroLib/CoordinateSystems/QUA2EUL ==
  note: Rotation representation
      |
      | Quaternion parameters to
      | Euler angles (rad)
  Quaternion : Inport  Port=1  LatchInput=off
  Axx3 : Fcn  Expr=u(1)*u(1) - u(2)*u(2) - u(3)*u(3) + u(4)*u(4)
  Axx4 : Fcn  Expr=u(1)*u(1) + u(2)*u(2) - u(3)*u(3) - u(4)*u(4)
  Axx5 : Fcn  Expr=2*(u(1)*u(2) + u(3)*u(4))
  Axx6 : Fcn  Expr=2*(u(1)*u(4) + u(2)*u(3))
  Azz3 : Fcn  Expr=2*(u(1)*u(3) - u(2)*u(4))
  Bound_2pi : Subsystem
  Bound_pi : Subsystem
  Bound_pi1 : Subsystem
  Mux1 : Mux  Inputs=3
  Trigonometric Function : Trigonometry  Operator=atan2
  Trigonometric Function1 : Trigonometry  Operator=atan2
  Trigonometric Function2 : Trigonometry  Operator=asin
  Euler : Outport  InitialOutput=0
  wires:
  Mux1/1 -> Euler/1
  Axx5/1 -> Trigonometric Function/1
  Axx3/1 -> Trigonometric Function/2
  Azz3/1 -> Trigonometric Function2/1
  Axx6/1 -> Trigonometric Function1/1
  Axx4/1 -> Trigonometric Function1/2
  Trigonometric Function/1 -> Bound_pi/1(In)  "Phi"
  Trigonometric Function1/1 -> Bound_2pi/1(In)  "Psi"
  Trigonometric Function2/1 -> Bound_pi1/1(In)  "Theta"
  Quaternion/1 -> Azz3/1, Axx5/1, Axx3/1, Axx4/1, Axx6/1
  Bound_pi/1(Out) -> Mux1/1  "Phi"
  Bound_pi1/1(Out) -> Mux1/2  "Theta"
  Bound_2pi/1(Out) -> Mux1/3  "Psi"

== system AeroLib/CoordinateSystems/STA2BOA ==
  note: Transformation from
      | Stability axes to
      | Body Axes
  Sta_In : Inport  Port=1  LatchInput=off
  Alpha_deg : Inport  Port=2  LatchInput=off
  Demux : Demux  Outputs=6
  Fcn : Fcn  Expr=-u(1)*u(8)+u(3)*u(7)
  Fcn1 : Fcn  Expr=-u(3)*u(8)-u(1)*u(7)
  Fcn2 : Fcn  Expr=u(4)*u(8)-u(6)*u(7)
  Fcn3 : Fcn  Expr=u(6)*u(8)+u(4)*u(7)
  Fcn4 : Fcn  Expr=u(2)
  Fcn5 : Fcn  Expr=u(5)
  Gain : Gain  Gain=pi/180  SaturateOnIntegerOverflow=on
  Mux : Mux  Inputs=8
  Mux1 : Mux  Inputs=6
  Trigonometric Function : Trigonometry
  Trigonometric Function1 : Trigonometry  Operator=cos
  Body_Out : Outport
  wires:
  Mux1/1 -> Body_Out/1
  Fcn4/1 -> Mux1/2  "Cy"
  Fcn5/1 -> Mux1/5  "CM"
  Trigonometric Function1/1 -> Mux/8
  Trigonometric Function/1 -> Mux/7
  Demux/5 -> Mux/5  "CMs"
  Demux/2 -> Mux/2  "CYs"
  Sta_In/1 -> Demux/1
  Fcn3/1 -> Mux1/6  "CN"
  Fcn2/1 -> Mux1/4  "CR"
  Fcn1/1 -> Mux1/3  "Cz"
  Fcn/1 -> Mux1/1  "Cx"
  Mux/1 -> Fcn5/1, Fcn3/1, Fcn2/1, Fcn4/1, Fcn/1, Fcn1/1
  Demux/6 -> Mux/6  "CNs"
  Demux/4 -> Mux/4  "CRs"
  Demux/3 -> Mux/3  "CLs"
  Demux/1 -> Mux/1  "CDs"
  Gain/1 -> Trigonometric Function1/1, Trigonometric Function/1
  Alpha_deg/1 -> Gain/1

== system AeroLib/CoordinateSystems/WND2STA ==
  note: Transformation from
      | Wind axes to
      | Stability axes
  Wind_In : Inport  Port=1  LatchInput=off
  Beta_deg : Inport  Port=2  LatchInput=off
  Deg-->Rad : Gain  Gain=pi/180  SaturateOnIntegerOverflow=on
  Fcn1 : Fcn  Expr=u(4)*u(8) - u(5)*u(7)*Geom.C_B
  Fcn2 : Fcn  Expr=u(1)*u(8) + u(2)*u(7)
  Fcn3 : Fcn  Expr=u(2)*u(8) - u(1)*u(7)
  Fcn4 : Fcn  Expr=u(5)*u(8) + u(4)*u(7)*Geom.B_C
  Fcn5 : Fcn  Expr=u(3)
  Fcn6 : Fcn  Expr=u(6)
  Mux : Mux  Inputs=3
  Mux2 : Mux  Inputs=6
  Trigonometric Function : Trigonometry
  Trigonometric Function1 : Trigonometry  Operator=cos
  Sta_Out : Outport
  wires:
  Beta_deg/1 -> Deg-->Rad/1
  Mux/1 -> Fcn3/1, Fcn2/1, Fcn5/1, Fcn1/1, Fcn4/1, Fcn6/1
  Wind_In/1 -> Mux/1
  Fcn2/1 -> Mux2/1  "CDs"
  Fcn3/1 -> Mux2/2  "CYs"
  Fcn5/1 -> Mux2/3  "CLs"
  Fcn1/1 -> Mux2/4  "CRs"
  Fcn4/1 -> Mux2/5  "CMs"
  Fcn6/1 -> Mux2/6  "CNs"
  Mux2/1 -> Sta_Out/1
  Deg-->Rad/1 -> Trigonometric Function/1, Trigonometric Function1/1
  Trigonometric Function/1 -> Mux/2
  Trigonometric Function1/1 -> Mux/3

== system AeroLib/EquationsOfMotion/Equations_of_Motion ==
  From_LGear : Inport  Port=1  LatchInput=off
  From_Aero : Inport  Port=2  LatchInput=off
  From_Prop : Inport  Port=3  LatchInput=off
  From_Mass : Inport  Port=4  LatchInput=off
  From_Reset : Inport  Port=5  LatchInput=off
  Bus Selector1 : BusSelector  DialogController=Simulink.DDGSource_Bus  OutputSignals=Xthrust,Ythrust,Zthrust,Lthrust,Mthrust,Nthrust
  Bus Selector2 : BusSelector  DialogController=Simulink.DDGSource_Bus  OutputSignals=Xaero,Yaero,Zaero,Laero,Maero,Naero
  Bus Selector3 : BusSelector  DialogController=Simulink.DDGSource_Bus  OutputSignals=Xground,Yground,Zground,Lground,Mground,Nground
  Bus Selector4 : BusSelector  DialogController=Simulink.DDGSource_Bus  OutputSignals=Weight,Inertia
  EQM Six-DOF : Subsystem
  EQM_Outputs : Subsystem
  External_Forces_and_Moments : AeroLib/EquationsOfMotion/External_Forces_and_Moments
  Mux1 : Mux  Inputs=6
  Mux2 : Mux  Inputs=6
  Mux3 : Mux  Inputs=6
  Selector : Selector  Elements=[3]  InputPortWidth=3
  Selector1 : Selector  Elements=[2]  InputPortWidth=3
  EQM_Out : Outport
  wires:
  Selector1/1 -> EQM_Outputs/17(Mext)
  Selector/1 -> EQM_Outputs/16(Zext)
  External_Forces_and_Moments/4 -> EQM_Outputs/18(NxNyNz)
  External_Forces_and_Moments/1 -> EQM_Outputs/1(AG_b)
  EQM Six-DOF/14(GeodHeight) -> EQM_Outputs/15(GeodHeight)
  EQM Six-DOF/13(Longitude) -> EQM_Outputs/14(Longitude)
  EQM Six-DOF/12(Latitude) -> EQM_Outputs/13(Latitude)
  EQM Six-DOF/11(Vb) -> EQM_Outputs/12(Vb)
  EQM Six-DOF/10(Rates_deg) -> EQM_Outputs/11(RatesDeg)
  EQM Six-DOF/9(Rates_rad) -> EQM_Outputs/10(RatesRad)
  EQM Six-DOF/8(Quaternion) -> EQM_Outputs/9(Quat)
  EQM Six-DOF/7(Euler_deg) -> EQM_Outputs/8(EulerDeg)
  EQM Six-DOF/6(Euler_rad) -> EQM_Outputs/7(EulerRad)
  EQM Six-DOF/5(Vel_NED) -> EQM_Outputs/6(Vel_NED)
  EQM Six-DOF/4(EulerDot_degps) -> EQM_Outputs/5(AttRates_Degps)
  EQM Six-DOF/3(Xe) -> EQM_Outputs/4(Xe)
  EQM Six-DOF/2(Ve) -> EQM_Outputs/3(Ve)
  EQM Six-DOF/1(DCM) -> External_Forces_and_Moments/1, EQM_Outputs/2(DCM)
  Bus Selector4/1 -> External_Forces_and_Moments/5, EQM Six-DOF/3(Weight)  "<Weight>"
  From_Mass/1 -> Bus Selector4/1
  EQM_Outputs/1(EQM_Out) -> EQM_Out/1
  Bus Selector1/3 -> Mux1/3  "<Zthrust>"
  Bus Selector1/6 -> Mux1/6  "<Nthrust>"
  Bus Selector1/5 -> Mux1/5  "<Mthrust>"
  Bus Selector1/4 -> Mux1/4  "<Lthrust>"
  Bus Selector1/2 -> Mux1/2  "<Ythrust>"
  Bus Selector1/1 -> Mux1/1  "<Xthrust>"
  Bus Selector2/6 -> Mux2/6  "<Naero>"
  Bus Selector2/5 -> Mux2/5  "<Maero>"
  Bus Selector2/4 -> Mux2/4  "<Laero>"
  Bus Selector2/3 -> Mux2/3  "<Zaero>"
  Bus Selector2/2 -> Mux2/2  "<Yaero>"
  Bus Selector2/1 -> Mux2/1  "<Xaero>"
  Mux2/1 -> External_Forces_and_Moments/3
  From_Aero/1 -> Bus Selector2/1
  Mux1/1 -> External_Forces_and_Moments/4
  From_Prop/1 -> Bus Selector1/1
  External_Forces_and_Moments/2 -> Selector/1, EQM Six-DOF/1(Forces X Y Z)
  External_Forces_and_Moments/3 -> Selector1/1, EQM Six-DOF/2(Moments L M N)
  Bus Selector4/2 -> EQM Six-DOF/4(Inertia)  "<Inertia>"
  Bus Selector3/1 -> Mux3/1  "<Xground>"
  Bus Selector3/6 -> Mux3/6  "<Nground>"
  Bus Selector3/5 -> Mux3/5  "<Mground>"
  Bus Selector3/4 -> Mux3/4  "<Lground>"
  Bus Selector3/3 -> Mux3/3  "<Zground>"
  Bus Selector3/2 -> Mux3/2  "<Yground>"
  From_LGear/1 -> Bus Selector3/1
  Mux3/1 -> External_Forces_and_Moments/2
  From_Reset/1 -> EQM Six-DOF/5(From_Reset)

== system AeroLib/EquationsOfMotion/External_Forces_and_Moments ==
  DCM : Inport  Port=1  LatchInput=off
  Fgear : Inport  Port=2  LatchInput=off
  Faero : Inport  Port=3  LatchInput=off
  Fthrust : Inport  Port=4  LatchInput=off
  Weight : Inport  Port=5  LatchInput=off
  Constant : Constant  Value=0
  Demux : Demux  Outputs=2
  Fcn : Fcn  Expr=u(1)/u(4)
  Fcn1 : Fcn  Expr=u(2)/u(4)
  Fcn2 : Fcn  Expr=-u(3)/u(4)
  Fcn3 : Fcn  Expr=u(1)/u(4)
  Fcn4 : Fcn  Expr=u(2)/u(4)
  Fcn5 : Fcn  Expr=u(3)/u(4)
  Mux : Mux  Inputs=3
  Mux1 : Mux  Inputs=2
  Mux2 : Mux  Inputs=3
  Mux3 : Mux  Inputs=2
  Mux4 : Mux  Inputs=3
  Sum : Sum  Inputs=+++  SaturateOnIntegerOverflow=on  InputSameDT=on
  Total Force : Sum  Inputs=|++  SaturateOnIntegerOverflow=on  InputSameDT=on
  Transpose : Math  Operator=transpose  SaturateOnIntegerOverflow=on
  Wxb Wyb Wzb : Product  Multiplication=Matrix(*)  SaturateOnIntegerOverflow=on  InputSameDT=on
  Ax_b Ay_b Az_b : Outport
  Fx_b Fy_b Fz_b : Outport  Port=2
  Mx_b My_b Mz_b : Outport  Port=3
  Nx_b Ny_b Nz_b : Outport  Port=4
  wires:
  Mux3/1 -> Fcn5/1, Fcn4/1, Fcn3/1
  Fcn3/1 -> Mux4/1
  Fcn4/1 -> Mux4/2
  Fcn5/1 -> Mux4/3
  Mux4/1 -> Ax_b Ay_b Az_b/1
  Faero/1 -> Sum/2
  Fthrust/1 -> Sum/3
  Total Force/1 -> Mux3/1, Fx_b Fy_b Fz_b/1
  Fgear/1 -> Sum/1
  Weight/1 -> Mux3/2, Mux1/2, Mux/3
  Mux/1 -> Wxb Wyb Wzb/2
  Wxb Wyb Wzb/1 -> Total Force/1
  Constant/1 -> Mux/2, Mux/1
  Sum/1 -> Demux/1
  DCM/1 -> Transpose/1
  Transpose/1 -> Wxb Wyb Wzb/1
  Mux1/1 -> Fcn/1, Fcn1/1, Fcn2/1
  Fcn/1 -> Mux2/1
  Fcn1/1 -> Mux2/2
  Fcn2/1 -> Mux2/3
  Mux2/1 -> Nx_b Ny_b Nz_b/1
  Demux/2 -> Mx_b My_b Mz_b/1
  Demux/1 -> Mux1/1, Total Force/2

== system AeroLib/GroundReactions/Gear_Out ==
  Bus Creator : BusCreator  DialogController=Simulink.DDGSource_Bus  Inputs=9
  Constant1 : Constant  Value=0
  Constant2 : Constant  Value=[0 0 0]
  Constant3 : Constant  Value=[0 0 0]
  Constant5 : Constant  Value=0
  Constant6 : Constant  Value=0
  Demux : Demux  Outputs=3
  Demux1 : Demux  Outputs=3
  GR_Out : Outport
  wires:
  Constant1/1 -> Bus Creator/7  "TireCompLmg"
  Constant5/1 -> Bus Creator/8  "TireCompNg"
  Constant6/1 -> Bus Creator/9  "TireCompRmg"
  Bus Creator/1 -> GR_Out/1
  Demux/1 -> Bus Creator/1  "Xground"
  Demux/2 -> Bus Creator/2  "Yground"
  Demux/3 -> Bus Creator/3  "Zground"
  Demux1/1 -> Bus Creator/4  "Lground"
  Demux1/2 -> Bus Creator/5  "Mground"
  Demux1/3 -> Bus Creator/6  "Nground"
  Constant2/1 -> Demux/1
  Constant3/1 -> Demux1/1

== system AeroLib/GroundReactions/Landing_Gear ==
  From_AP : Inport  Port=1  LatchInput=off
  From_Inputs : Inport  Port=2  LatchInput=off
  From_EQM : Inport  Port=3  LatchInput=off
  Bus Selector : BusSelector  DialogController=Simulink.DDGSource_Bus  OutputSignals=Brake,NoseWheel
  Bus Selector1 : BusSelector  DialogController=Simulink.DDGSource_Bus  OutputSignals=Vb,P_rad,Q_rad,R_rad,DCM,Phi_rad,The_rad,Psi_rad,Hagl_m
  Bus Selector2 : BusSelector  DialogController=Simulink.DDGSource_Bus  OutputSignals=AP_Brake,AP_Caster
  GHM Dir_Cos : Subsystem
  GHM Ground_Reactions : Subsystem
  Left Main Gear Dynamics : Subsystem  mask{CFriction=Lgear(1).Strut.CFriction, Mass=Lgear(1).Mass, Strut_Deflection=Lgear(1).Strut.Deflection, Strut_Stiffness=Lgear(1).Strut.Stiffness, Damping=Lgear(1).Strut.Damping, Strut_Limit=Lgear(1).Strut.Limit, TireMaxComp=Lgear(1).Tire.MaxComp, Tire_Stiffness=Lgear(1).Tire.Stiffness, AccFactor=Lgear(1).Strut.AccFactor}
      mask prompts: CFriction "Coulomb Friction"; Mass "Landing Gear Mass"; Strut_Deflection "Strut Deflection"; Strut_Stiffness "Strut Stiffness"; Damping "Strut Damping"; Strut_Limit "Strut Limit"; TireMaxComp "Tire Max Compression"; Tire_Stiffness "Tire Stiffness"; AccFactor "Acc Factor"
  Nose Gear Dynamics : Subsystem  mask{CFriction=Lgear(2).Strut.CFriction, Mass=Lgear(2).Mass, Strut_Deflection=Lgear(2).Strut.Deflection, Strut_Stiffness=Lgear(2).Strut.Stiffness, Damping=Lgear(2).Strut.Damping, Strut_Limit=Lgear(2).Strut.Limit, TireMaxComp=Lgear(2).Tire.MaxComp, Tire_Stiffness=Lgear(2).Tire.Stiffness, AccFactor=Lgear(2).Strut.AccFactor}
      mask prompts: CFriction "Coulomb Friction"; Mass "Landing Gear Mass"; Strut_Deflection "Strut Deflection"; Strut_Stiffness "Strut Stiffness"; Damping "Strut Damping"; Strut_Limit "Strut Limit"; TireMaxComp "Tire Max Compression"; Tire_Stiffness "Tire Stiffness"; AccFactor "Acc Factor"
  Right Main Gear Dynamics : Subsystem  mask{CFriction=Lgear(1).Strut.CFriction, Mass=Lgear(1).Mass, Strut_Deflection=Lgear(1).Strut.Deflection, Strut_Stiffness=Lgear(1).Strut.Stiffness, Damping=Lgear(1).Strut.Damping, Strut_Limit=Lgear(1).Strut.Limit, TireMaxComp=Lgear(1).Tire.MaxComp, Tire_Stiffness=Lgear(1).Tire.Stiffness, AccFactor=Lgear(1).Strut.AccFactor}
      mask prompts: CFriction "Coulomb Friction"; Mass "Landing Gear Mass"; Strut_Deflection "Strut Deflection"; Strut_Stiffness "Strut Stiffness"; Damping "Strut Damping"; Strut_Limit "Strut Limit"; TireMaxComp "Tire Max Compression"; Tire_Stiffness "Tire Stiffness"; AccFactor "Acc Factor"
  Sum : Sum  Inputs=|++  SaturateOnIntegerOverflow=on  InputSameDT=on
  LGear_Out : Outport
  wires:
  GHM Dir_Cos/10(Conf_Tire_RposRmg) -> Right Main Gear Dynamics/6(Conf_Tire_RposRmg)
  GHM Dir_Cos/9(Conf_Tire_RposNg) -> Nose Gear Dynamics/5(Conf_Tire_RposNg)
  GHM Dir_Cos/8(Conf_Tire_RposLmg) -> Left Main Gear Dynamics/6(Conf_Tire_RposLmg)
  GHM Dir_Cos/3(DCbg) -> Nose Gear Dynamics/3(DCbg), Right Main Gear Dynamics/4(DCbg), Left Main Gear Dynamics/4(DCbg)  "DCbg"
  GHM Dir_Cos/6(HaglLmg) -> Left Main Gear Dynamics/5(Hagl)  "HAGL_LMG"
  GHM Dir_Cos/1(VelB) -> Left Main Gear Dynamics/2(VelB), Nose Gear Dynamics/1(VelB), Right Main Gear Dynamics/2(VelB)  "VelB"
  GHM Dir_Cos/2(RatesB) -> Left Main Gear Dynamics/3(RatesB), Nose Gear Dynamics/2(RatesB), Right Main Gear Dynamics/3(RatesB)  "RatesB"
  GHM Dir_Cos/5(HaglNg) -> Nose Gear Dynamics/4(Hagl)  "HAGL_NG"
  GHM Dir_Cos/7(HaglRmg) -> Right Main Gear Dynamics/5(Hagl)  "HAGL_RMG"
  Left Main Gear Dynamics/1(MUeff) -> GHM Ground_Reactions/1(MUeLmg)
  Left Main Gear Dynamics/2(MUside) -> GHM Ground_Reactions/2(MUsLmg)
  Left Main Gear Dynamics/3(TireForce) -> GHM Ground_Reactions/3(FstrLmg)
  Left Main Gear Dynamics/4(Rtb) -> GHM Ground_Reactions/4(Rlmg)
  Nose Gear Dynamics/1(MUeff) -> GHM Ground_Reactions/6(MUeNg)
  Nose Gear Dynamics/2(MUside) -> GHM Ground_Reactions/7(MUsNg)
  Nose Gear Dynamics/3(TireForce) -> GHM Ground_Reactions/8(FstrNg)
  Nose Gear Dynamics/4(Rtb) -> GHM Ground_Reactions/9(Rng)
  Right Main Gear Dynamics/1(MUeff) -> GHM Ground_Reactions/13(MUeRmg)
  Right Main Gear Dynamics/3(TireForce) -> GHM Ground_Reactions/15(FstrRmg)
  Right Main Gear Dynamics/4(Rtb) -> GHM Ground_Reactions/16(Rrmg)
  Nose Gear Dynamics/5(TireComp) -> GHM Ground_Reactions/10(TireCompNg)
  Left Main Gear Dynamics/5(TireComp) -> GHM Ground_Reactions/5(TireCompLmg)
  Right Main Gear Dynamics/5(TireComp) -> GHM Ground_Reactions/17(TireCompRmg)
  GHM Ground_Reactions/1(GR_Out) -> LGear_Out/1
  Bus Selector2/2 -> Nose Gear Dynamics/6(Caster)  "<AP_Caster>"
  From_Inputs/1 -> Bus Selector/1
  Bus Selector/2 -> Nose Gear Dynamics/7(NoseWheel)  "<NoseWheel>"
  From_EQM/1 -> Bus Selector1/1
  From_AP/1 -> Bus Selector2/1
  Bus Selector2/1 -> Sum/2  "<AP_Brake>"
  Bus Selector/1 -> Sum/1  "<Brake>"
  Sum/1 -> Left Main Gear Dynamics/1(Brake), Right Main Gear Dynamics/1(Brake)
  Right Main Gear Dynamics/2(MUside) -> GHM Ground_Reactions/14(MUsRmg)
  Bus Selector1/1 -> GHM Dir_Cos/1(Vb)  "<Vb>"
  Bus Selector1/2 -> GHM Dir_Cos/2(Prate)  "<P_rad>"
  Bus Selector1/3 -> GHM Dir_Cos/3(Qrate)  "<Q_rad>"
  Bus Selector1/4 -> GHM Dir_Cos/4(Rrate)  "<R_rad>"
  Bus Selector1/5 -> GHM Dir_Cos/5(DCM)  "<DCM>"
  Bus Selector1/9 -> GHM Dir_Cos/9(Hagl)  "<Hagl_m>"
  Bus Selector1/6 -> GHM Dir_Cos/6(PhiRad)  "<Phi_rad>"
  Bus Selector1/7 -> GHM Dir_Cos/7(ThetaRad)  "<The_rad>"
  Bus Selector1/8 -> GHM Dir_Cos/8(PsiRad)  "<Psi_rad>"
  GHM Dir_Cos/4(EulerRad) -> GHM Ground_Reactions/12(EulerRad)
  Nose Gear Dynamics/6(NoseWheelAng) -> GHM Ground_Reactions/11(NoseWheelAng)

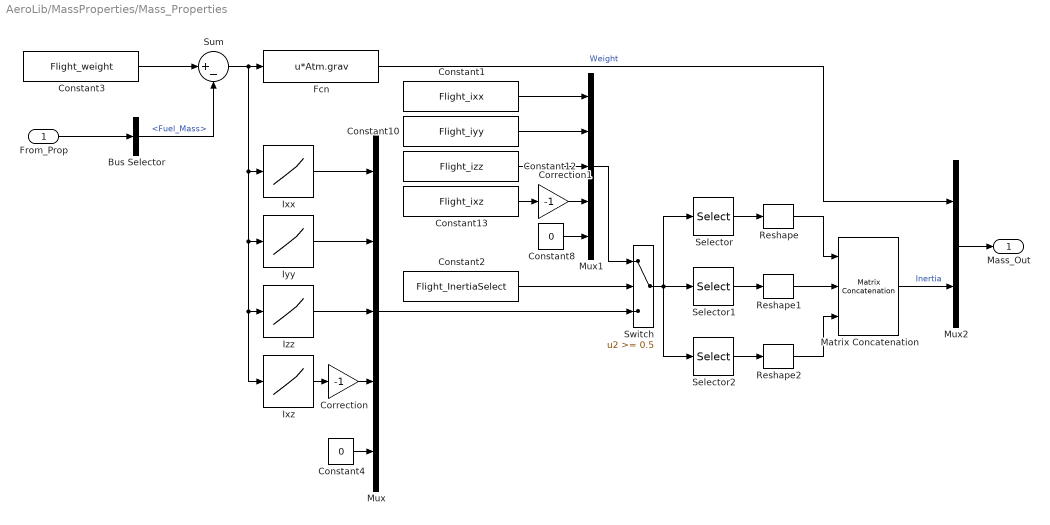
== system AeroLib/MassProperties/Mass_Properties ==
  From_Prop : Inport  Port=1  LatchInput=off
  Bus Selector : BusSelector  DialogController=Simulink.DDGSource_Bus  OutputSignals=Fuel_Mass
  Constant1 : Constant  Value=Flight_ixx
  Constant10 : Constant  Value=Flight_iyy
  Constant12 : Constant  Value=Flight_izz
  Constant13 : Constant  Value=Flight_ixz
  Constant2 : Constant  Value=Flight_InertiaSelect
  Constant3 : Constant  Value=Flight_weight
  Constant4 : Constant  Value=0
  Constant8 : Constant  Value=0
  Correction : Gain  Gain=-1  SaturateOnIntegerOverflow=on
  Correction1 : Gain  Gain=-1  SaturateOnIntegerOverflow=on
  Fcn : Fcn  Expr=u*Atm.grav
  Ixx : Lookup  DialogController=Simulink.DDGSource  InputValues=Mass.Iweight  OutputValues=Mass.Ixx  SaturateOnIntegerOverflow=on
  Ixz : Lookup  DialogController=Simulink.DDGSource  InputValues=Mass.Iweight  OutputValues=Mass.Ixz  SaturateOnIntegerOverflow=on
  Iyy : Lookup  DialogController=Simulink.DDGSource  InputValues=Mass.Iweight  OutputValues=Mass.Iyy  SaturateOnIntegerOverflow=on
  Izz : Lookup  DialogController=Simulink.DDGSource  InputValues=Mass.Iweight  OutputValues=Mass.Izz  SaturateOnIntegerOverflow=on
  Matrix Concatenation : simulink3/Signals & Systems/Matrix Concatenation  numInports=3  catMethod=Vertical
  Mux : Mux  Inputs=5
  Mux1 : Mux  Inputs=5
  Mux2 : Mux  Inputs=2
  Reshape : simulink3/Signals & Systems/Reshape  OutputDimensionality=Row vector  OutputDimensions=[1,1]
  Reshape1 : simulink3/Signals & Systems/Reshape  OutputDimensionality=Row vector  OutputDimensions=[1,1]
  Reshape2 : simulink3/Signals & Systems/Reshape  OutputDimensionality=Row vector  OutputDimensions=[1,1]
  Selector : Selector  Elements=[1 5 4]  InputPortWidth=5
  Selector1 : Selector  Elements=[5 2 5]  InputPortWidth=5
  Selector2 : Selector  Elements=[4 5 3]  InputPortWidth=5
  Sum : Sum  Inputs=|+-  SaturateOnIntegerOverflow=on  InputSameDT=on
  Switch : Switch  Threshold=0.5  SaturateOnIntegerOverflow=on  InputSameDT=on
  Mass_Out : Outport
  wires:
  Fcn/1 -> Mux2/1  "Weight"
  Mux2/1 -> Mass_Out/1
  Reshape2/1 -> Matrix Concatenation/3
  Reshape1/1 -> Matrix Concatenation/2
  Reshape/1 -> Matrix Concatenation/1
  Matrix Concatenation/1 -> Mux2/2  "Inertia"
  Selector2/1 -> Reshape2/1
  Selector1/1 -> Reshape1/1
  Selector/1 -> Reshape/1
  Constant4/1 -> Mux/5
  Ixz/1 -> Correction/1
  Izz/1 -> Mux/3
  Iyy/1 -> Mux/2
  Ixx/1 -> Mux/1
  Constant2/1 -> Switch/2
  Constant13/1 -> Correction1/1
  Constant12/1 -> Mux1/3
  Constant10/1 -> Mux1/2
  Constant1/1 -> Mux1/1
  Constant8/1 -> Mux1/5
  Switch/1 -> Selector/1, Selector2/1, Selector1/1
  Mux/1 -> Switch/3
  Mux1/1 -> Switch/1
  Correction/1 -> Mux/4
  Correction1/1 -> Mux1/4
  Constant3/1 -> Sum/1
  From_Prop/1 -> Bus Selector/1
  Bus Selector/1 -> Sum/2  "<Fuel_Mass>"
  Sum/1 -> Fcn/1, Ixx/1, Iyy/1, Izz/1, Ixz/1

== system AeroLib/Propulsion/Booster ==
  Booster_ON : Inport  Port=1  LatchInput=off
  From_Reset : Inport  Port=2  LatchInput=off
  3x3 cross product : aerospace/Axes Transformations/3x3 cross product
  AverThrustBooster_N : Constant  Value=Booster_Thrust
  BoosterTime : Fcn  Expr=u >= Booster_Time
  Clock4 : Clock
      settings: Decimation=10
  Constant3 : Constant  Value=[Xpos Ypos Zpos]
  Fcn1 : Fcn  Expr=1-u
  Fcn2 : Fcn  Expr=u == 0
  Fcn3 : Fcn  Expr=u <= 0.1
  Fthrust_Booster : Subsystem
  Logical Operator1 : Logic
  Logical Operator2 : Logic
  Mem : Memory
  Mux1 : Mux  Inputs=2
  Product : Product  Inputs=3  SaturateOnIntegerOverflow=on  InputSameDT=on
  Sum1 : Sum  Inputs=|+-  SaturateOnIntegerOverflow=on  InputSameDT=on
  Sw4 : Switch  Threshold=0.5  SaturateOnIntegerOverflow=on  InputSameDT=on
  Thrust : Subsystem
  Booster_Out : Outport
  StopBooster : Outport  Port=2
  wires:
  BoosterTime/1 -> Logical Operator1/1
  Logical Operator1/1 -> Fcn1/1, Logical Operator2/1
  Booster_ON/1 -> Fcn2/1, Logical Operator1/2, Product/3
  Fcn2/1 -> Sw4/2
  Sum1/1 -> BoosterTime/1  "TimeAfterBoosterStart"
  Sw4/1 -> Mem/1, Sum1/2
  Mem/1 -> Sw4/3
  Fcn1/1 -> Product/2
  AverThrustBooster_N/1 -> Product/1
  Constant3/1 -> 3x3 cross product/1
  3x3 cross product/1 -> Mux1/2
  Mux1/1 -> Booster_Out/1
  Fthrust_Booster/1(LHFthr) -> Mux1/1, 3x3 cross product/2
  Product/1 -> Thrust/1(In1)
  Thrust/1(Out1) -> Fthrust_Booster/1(LH NT), Fcn3/1
  Logical Operator2/1 -> StopBooster/1
  Fcn3/1 -> Logical Operator2/2
  From_Reset/1 -> Thrust/2(From_Reset)
  Clock4/1 -> Sum1/1, Sw4/1

== system AeroLib/Propulsion/Engine_Empty ==
  Bus Creator : BusCreator  DialogController=Simulink.DDGSource_Bus  Inputs=16
  Constant{,2..15} (15 alike) : Constant  Value=0
  Constant1 : Constant  Value=Xthrust
  Prop_Out : Outport
  wires:
  Constant14/1 -> Bus Creator/14  "RH_Throttle"
  Constant6/1 -> Bus Creator/13  "LH_Throttle"
  Constant5/1 -> Bus Creator/11  "Thrust_N"
  Constant13/1 -> Bus Creator/12  "DeltaThr"
  Constant12/1 -> Bus Creator/10  "Thrust_Kgf"
  Constant4/1 -> Bus Creator/9  "CT"
  Constant11/1 -> Bus Creator/8  "Nthrust"
  Constant3/1 -> Bus Creator/7  "Mthrust"
  Bus Creator/1 -> Prop_Out/1
  Constant1/1 -> Bus Creator/3  "Xthrust"
  Constant10/1 -> Bus Creator/6  "Lthrust"
  Constant2/1 -> Bus Creator/5  "Zthrust"
  Constant9/1 -> Bus Creator/4  "Ythrust"
  Constant15/1 -> Bus Creator/16  "StopBooster"
  Constant7/1 -> Bus Creator/15  "Fuel_Mass"
  Constant/1 -> Bus Creator/1  "Rpm_Eng"
  Constant8/1 -> Bus Creator/2  "Effic_Prop"

== system AeroLib/Propulsion/Engine_Transient ==
  From_Ctrl : Inport  Port=1  LatchInput=off
  From_Reset : Inport  Port=2  LatchInput=off
  Bus Selector1 : BusSelector  DialogController=Simulink.DDGSource_Bus  OutputSignals=Thr_LH,Thr_RH
  Engine_Transient_LH : Subsystem
  Engine_Transient_RH : Subsystem
  Throttle_LH : Outport
  Throttle_RH : Outport  Port=2
  wires:
  Engine_Transient_RH/1(TLA) -> Throttle_RH/1
  Engine_Transient_LH/1(TLA) -> Throttle_LH/1
  Bus Selector1/1 -> Engine_Transient_LH/1(Throttle)  "<Thr_LH>"
  Bus Selector1/2 -> Engine_Transient_RH/1(Throttle)  "<Thr_RH>"
  From_Ctrl/1 -> Bus Selector1/1
  From_Reset/1 -> Engine_Transient_LH/2(From_Reset), Engine_Transient_RH/2(From_Reset)

== system AeroLib/Propulsion/Fixed_Pitch_Propeller ==
  RPM : Inport  Port=1  LatchInput=off
  Mach : Inport  Port=2  LatchInput=off
  TAS_mps : Inport  Port=3  LatchInput=off
  Advance_Ratio : Fcn  Expr=u(1)/(prop_diam*u(2))
  CP : simulink/Lookup Tables/Interpolation (n-D) using PreLookup  numDimsPopupSelect=1  explicitNumDims=2  table=Eng.Prop.Cp  interpMethod=Linear  extrapMethod=Linear  rangeErrorMode=None  NumSelectionDims=0
  CT : simulink/Lookup Tables/Interpolation (n-D) using PreLookup  numDimsPopupSelect=1  explicitNumDims=2  table=Eng.Prop.Ct  interpMethod=Linear  extrapMethod=Linear  rangeErrorMode=None  NumSelectionDims=0
  J : simulink/Lookup Tables/PreLookup Index Search  bpData=Eng.Prop.J  searchMode=Binary Search  cacheBpFlag=off  outputFlag=off  IndexDataType=uint32  extrapMode=Linear Extrapolation  rangeErrorMode=None
  Mach_Number_Effect : Subsystem
  Mux1 : Mux  Inputs=2
  Product1 : Product  Inputs=**/  SaturateOnIntegerOverflow=on  InputSameDT=on
  Product2 : Product  Inputs=*/  SaturateOnIntegerOverflow=on  InputSameDT=on
  Product4 : Product  SaturateOnIntegerOverflow=on  InputSameDT=on
  Reduction : Gain  Gain=1/reduc/60  SaturateOnIntegerOverflow=on
  Thrust_coef : Outport
  Power_coef : Outport  Port=2
  Propeller_rps : Outport  Port=3
  Efficiency_coef : Outport  Port=4
  wires:
  J/1 -> CT/1, CP/1
  Mux1/1 -> Advance_Ratio/1
  CP/1 -> Product2/1
  Reduction/1 -> Mux1/2, Propeller_rps/1, Mach_Number_Effect/2(Prop_rps)
  TAS_mps/1 -> Mux1/1, Mach_Number_Effect/3(TAS)
  RPM/1 -> Reduction/1
  Product1/1 -> Efficiency_coef/1
  Mach/1 -> Mach_Number_Effect/4(Mach)
  Product2/1 -> Power_coef/1, Product1/3
  Mach_Number_Effect/2(Kcp) -> Product2/2
  CT/1 -> Product4/1
  Product4/1 -> Product1/1, Thrust_coef/1
  Mach_Number_Effect/1(Km) -> Product4/2
  Advance_Ratio/1 -> Product1/2, J/1, Mach_Number_Effect/1(J)

== system AeroLib/Propulsion/Jet_Engine ==
  Throttle_In : Inport  Port=1  LatchInput=off
  From_Atmos : Inport  Port=2  LatchInput=off
  Fuel_Cut : Inport  Port=3  LatchInput=off
  From_Reset : Inport  Port=4  LatchInput=off
  Bus Selector2 : BusSelector  DialogController=Simulink.DDGSource_Bus  OutputSignals=Mach,PresAlt_ft
  Engine_Tables : Subsystem
  Terminator1 : Terminator
  Terminator2 : Terminator
  lbf--->N : Gain  Gain=4.448222  SaturateOnIntegerOverflow=on
  NetThrust_N : Outport
  Fuel_Mass : Outport  Port=2
  Throttle : Outport  Port=3
  wires:
  Fuel_Cut/1 -> Engine_Tables/5(FuelCut)
  Throttle_In/1 -> Engine_Tables/1(TRA), Throttle/1
  Engine_Tables/1(GrossThrust) -> Terminator1/1
  Engine_Tables/2(NetThrust) -> lbf--->N/1
  Engine_Tables/3(RamDrag) -> Terminator2/1
  lbf--->N/1 -> NetThrust_N/1
  Bus Selector2/1 -> Engine_Tables/2(Mach)  "<Mach>"
  Bus Selector2/2 -> Engine_Tables/3(Alt)  "<PresAlt_ft>"
  From_Atmos/1 -> Bus Selector2/1
  Engine_Tables/4(Fuel_Mass) -> Fuel_Mass/1
  From_Reset/1 -> Engine_Tables/4(From_Reset)
